simulink model "Ejercicio_1"  (R2023b)
settings: Solver=VariableStepAuto  StartTime=0.0  StopTime=30  RelTol=1e-3
values from neighbouring files (symbols this model uses):
  a = 200    [parametros_auto.m]
  ang = 2    [parametros_auto.m]
  b = 10000    [parametros_auto.m]
  g = 9.81    [parametros_auto.m]
  ki = 20    [parametros_auto.m]
  kp = 60    [parametros_auto.m]
  m = 1000    [parametros_auto.m]
  m2 = 1500    [parametros_auto.m]
settings Model: Creator=tomas  LastModifiedBy=tomas

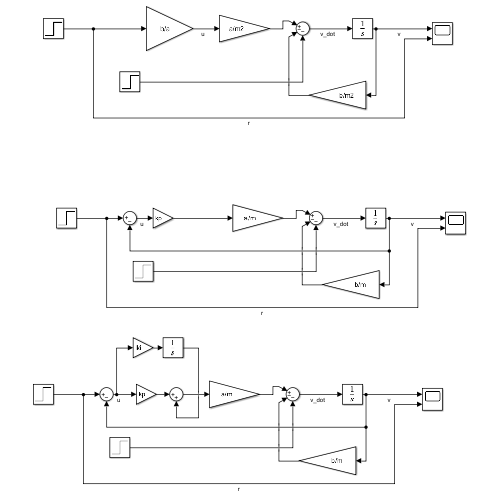
[thumbnail: Simulink's stored preview of the top-level diagram]
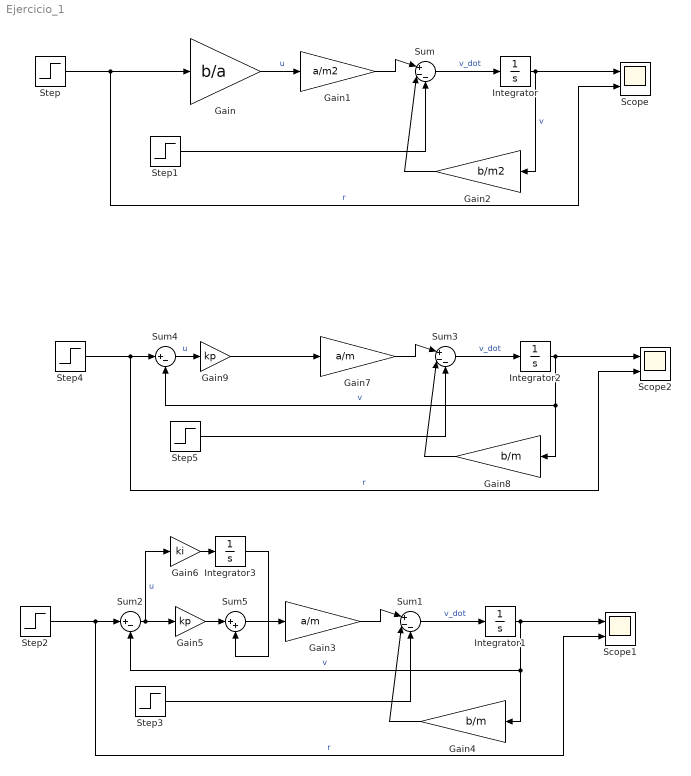
== system Ejercicio_1 ==
  Gain : Gain  Gain=b/a
  Gain1 : Gain  Gain=a/m2
  Gain2 : Gain  Gain=b/m2
  Gain3 : Gain  Gain=a/m
  Gain4 : Gain  Gain=b/m
  Gain5 : Gain  Gain=kp
  Gain6 : Gain  Gain=ki
  Gain7 : Gain  Gain=a/m
  Gain8 : Gain  Gain=b/m
  Gain9 : Gain  Gain=kp
  Integrator{,1..3} (4 alike) : Integrator
  Scope : Scope  NumInputPorts=2
  Scope1 : Scope  NumInputPorts=2
  Scope2 : Scope  NumInputPorts=2
  Step : Step  Time=10  Before=25  After=30  SampleTime=0
  Step1 : Step  Time=20  After=g*sin((ang/360)*2*pi)  SampleTime=0
  Step2 : Step  Time=10  Before=25  After=30  SampleTime=0
  Step3 : Step  Time=20  After=g*sin((ang/360)*2*pi)  SampleTime=0
  Step4 : Step  Time=10  Before=25  After=30  SampleTime=0
  Step5 : Step  Time=20  After=g*sin((ang/360)*2*pi)  SampleTime=0
  Sum : Sum  Inputs=|+--
  Sum1 : Sum  Inputs=|+--
  Sum2 : Sum  Inputs=|+-
  Sum3 : Sum  Inputs=|+--
  Sum4 : Sum  Inputs=|+-
  Sum5 : Sum  Inputs=|++
  wires:
  Step/1 -> Scope/2, Gain/1  "r"
  Gain/1 -> Gain1/1  "u"
  Gain1/1 -> Sum/1
  Sum/1 -> Integrator/1  "v_dot"
  Integrator/1 -> Gain2/1, Scope/1  "v"
  Gain2/1 -> Sum/2
  Step1/1 -> Sum/3
  Step5/1 -> Sum3/3
  Step4/1 -> Sum4/1, Scope2/2  "r"
  Gain7/1 -> Sum3/1
  Integrator2/1 -> Sum4/2, Gain8/1, Scope2/1  "v"
  Gain8/1 -> Sum3/2
  Sum3/1 -> Integrator2/1  "v_dot"
  Sum4/1 -> Gain9/1  "u"
  Gain9/1 -> Gain7/1
  Step3/1 -> Sum1/3
  Gain4/1 -> Sum1/2
  Gain3/1 -> Sum1/1
  Integrator1/1 -> Sum2/2, Gain4/1, Scope1/1  "v"
  Step2/1 -> Sum2/1, Scope1/2  "r"
  Sum2/1 -> Gain6/1, Gain5/1  "u"
  Sum1/1 -> Integrator1/1  "v_dot"
  Gain5/1 -> Sum5/1
  Sum5/1 -> Gain3/1
  Gain6/1 -> Integrator3/1
  Integrator3/1 -> Sum5/2
